simulink model "VMC_Controller"  (R2017b)
settings: Solver=VariableStepAuto  StartTime=0.0  StopTime=10.0  RelTol=1e-3
settings Model: Creator=Kalana  LastModifiedBy=Kalana

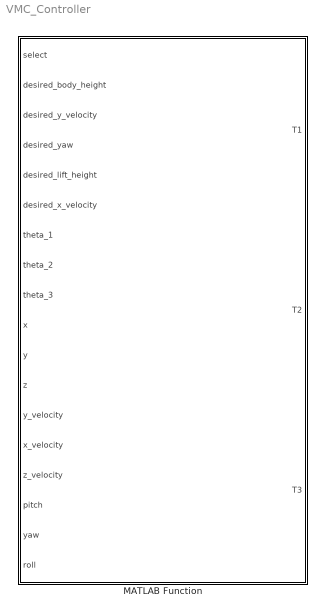
== system VMC_Controller ==
  MATLAB Function : MATLAB Function  TreatAsAtomicUnit=on

== matlab function VMC_Controller/MATLAB Function ==
  data: select input; T1 output; T2 output; T3 output; desired_body_height input; desired_y_velocity input; desired_yaw input; desired_lift_height input; desired_x_velocity input; theta_1 input; theta_2 input; theta_3 input; x input; y input; z input; y_velocity input; x_velocity input; z_velocity input; pitch input; yaw input; roll input
function [T1, T2, T3] = VMC_Controller(select, desired_body_height, desired_y_velocity, desired_yaw, desired_lift_height, desired_x_velocity, theta_1, theta_2, theta_3, x, y, z, y_velocity, x_velocity, z_velocity, pitch, yaw, roll)



y = u;
